simulink model "model_podstawowy_swingup_2015a"  (R2019b)
settings: Solver=ode45  StartTime=0.0  StopTime=15  RelTol=1e-3
undefined symbols (not defined in the file): g, J, K_reg, L, m, M, Q2, theta, x, x_konc, x_pocz
libraries: simulink x8
settings Model: Creator=maelstro  LastModifiedBy=Czarek
settings OptimizationCC: LifeSpan=inf
settings DebuggingCC: SFExecutionAtInitializationDiag=none  ArithmeticOperatorsInVariantConditions=warning
settings HardwareCC: ProdBitPerSizeT=32  ProdBitPerPtrDiffT=32  ProdWordSize=32  ProdHWDeviceType=Specified
settings SFSimCC: CustomCodeUndefinedFunction=UseInterfaceOnly
settings CodeAppCC: StateflowObjectComments=on

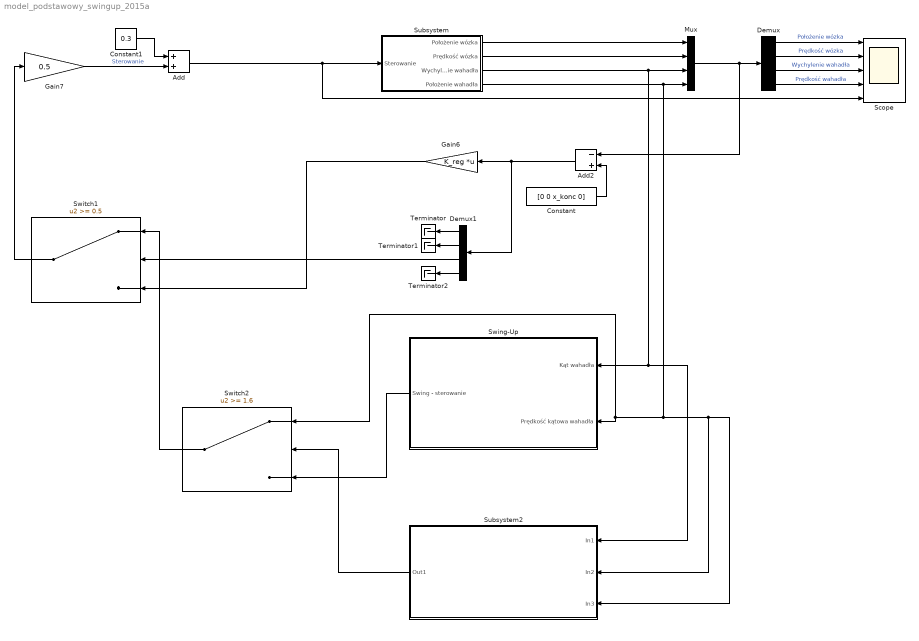
== system model_podstawowy_swingup_2015a ==
  Add : Sum
  Add2 : Sum  Inputs=-+
  Constant : Constant  Value=[0 0 x_konc 0]
  Constant1 : Constant  Value=0.3
  Demux : Demux
  Demux1 : Demux
  Gain6 : Gain  Gain=K_reg  Multiplication=Matrix(K*u)
  Gain7 : Gain  Gain=0.5
  Mux : Mux
  Scope : Scope  NumInputPorts=5
  Subsystem : Subsystem
  Subsystem2 : Subsystem
  Swing-Up : Subsystem
  Switch1 : Switch  Threshold=0.5
  Switch2 : Switch  Threshold=1.6
  Terminator : Terminator
  Terminator1 : Terminator
  Terminator2 : Terminator
  wires:
  Add2/1 -> Demux1/1, Gain6/1
  Mux/1 -> Demux/1, Add2/1
  Constant/1 -> Add2/2
  Subsystem/1(Położenie wózka) -> Mux/1
  Subsystem/2(Prędkość wózka) -> Mux/2
  Demux/1 -> Scope/1  "Położenie wózka"
  Demux/2 -> Scope/2  "Prędkość wózka"
  Demux/3 -> Scope/3  "Wychylenie wahadła"
  Demux/4 -> Scope/4  "Prędkość wahadła"
  Subsystem/4(Położenie wahadła) -> Switch2/1, Swing-Up/2(Prędkość kątowa wahadła), Subsystem2/3(In3), Subsystem2/2(In2), Mux/4
  Subsystem2/1(Out1) -> Switch2/2
  Switch2/1 -> Switch1/1
  Gain6/1 -> Switch1/3
  Subsystem/3(Wychylenie wahadła) -> Swing-Up/1(Kąt wahadła), Subsystem2/1(In1), Mux/3
  Swing-Up/1(Swing - sterowanie) -> Switch2/3
  Demux1/4 -> Terminator2/1
  Demux1/2 -> Terminator1/1
  Demux1/1 -> Terminator/1
  Demux1/3 -> Switch1/2
  Switch1/1 -> Gain7/1
  Gain7/1 -> Add/2  "Sterowanie"
  Add/1 -> Scope/5, Subsystem/1(Sterowanie)
  Constant1/1 -> Add/1

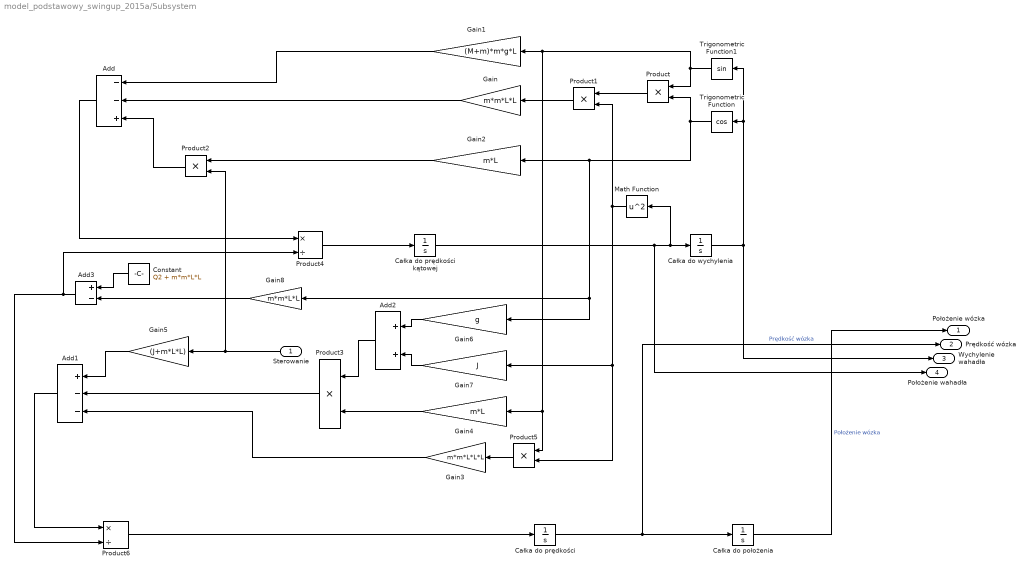
== system model_podstawowy_swingup_2015a/Subsystem ==
  Sterowanie : Inport
  Add : Sum  Inputs=--+
  Add1 : Sum  Inputs=+--
  Add2 : Sum
  Add3 : Sum  Inputs=+-
  Całka do położenia : Integrator
  Całka do prędkości : Integrator
  Całka do prędkości kątowej : Integrator
  Całka do wychylenia : Integrator  InitialCondition=x_pocz
  Constant : Constant  Value=Q2 + m*m*L*L
  Gain : Gain  Gain=m*m*L*L
  Gain1 : Gain  Gain=(M+m)*m*g*L
  Gain2 : Gain  Gain=m*L
  Gain3 : Gain  Gain=m*m*L*L*L
  Gain4 : Gain  Gain=m*L
  Gain5 : Gain  Gain=(J+m*L*L)
  Gain6 : Gain  Gain=g
  Gain7 : Gain  Gain=J
  Gain8 : Gain  Gain=m*m*L*L
  Math Function : Math  Operator=square  SaturateOnIntegerOverflow=on
  Product{,1..3,5} (5 alike) : Product
  Product4 : Product  Inputs=*/
  Product6 : Product  Inputs=*/
  Trigonometric Function : Trigonometry  Operator=cos
  Trigonometric Function1 : Trigonometry
  Położenie wózka : Outport
  Prędkość wózka : Outport  Port=2
  Wychylenie wahadła : Outport  Port=3
  Położenie wahadła : Outport  Port=4
  wires:
  Add/1 -> Product4/1
  Całka do prędkości/1 -> Prędkość wózka/1, Całka do położenia/1  "Prędkość wózka"
  Gain4/1 -> Product3/2
  Sterowanie/1 -> Product2/2, Gain5/1
  Product3/1 -> Add1/2
  Trigonometric Function/1 -> Gain8/1, Gain6/1, Gain2/1, Product/2
  Gain2/1 -> Product2/1
  Product1/1 -> Gain/1
  Całka do wychylenia/1 -> Wychylenie wahadła/1, Trigonometric Function1/1, Trigonometric Function/1
  Całka do położenia/1 -> Położenie wózka/1  "Położenie wózka"
  Add1/1 -> Product6/1
  Trigonometric Function1/1 -> Product/1, Product5/1, Gain4/1, Gain1/1
  Product4/1 -> Całka do prędkości kątowej/1
  Gain/1 -> Add/2
  Gain1/1 -> Add/1
  Product/1 -> Product1/1
  Product2/1 -> Add/3
  Gain3/1 -> Add1/3
  Całka do prędkości kątowej/1 -> Położenie wahadła/1, Math Function/1, Całka do wychylenia/1
  Gain5/1 -> Add1/1
  Math Function/1 -> Product1/2, Product5/2, Gain7/1
  Gain7/1 -> Add2/2
  Gain6/1 -> Add2/1
  Add2/1 -> Product3/1
  Product5/1 -> Gain3/1
  Product6/1 -> Całka do prędkości/1
  Add3/1 -> Product4/2, Product6/2
  Constant/1 -> Add3/1
  Gain8/1 -> Add3/2

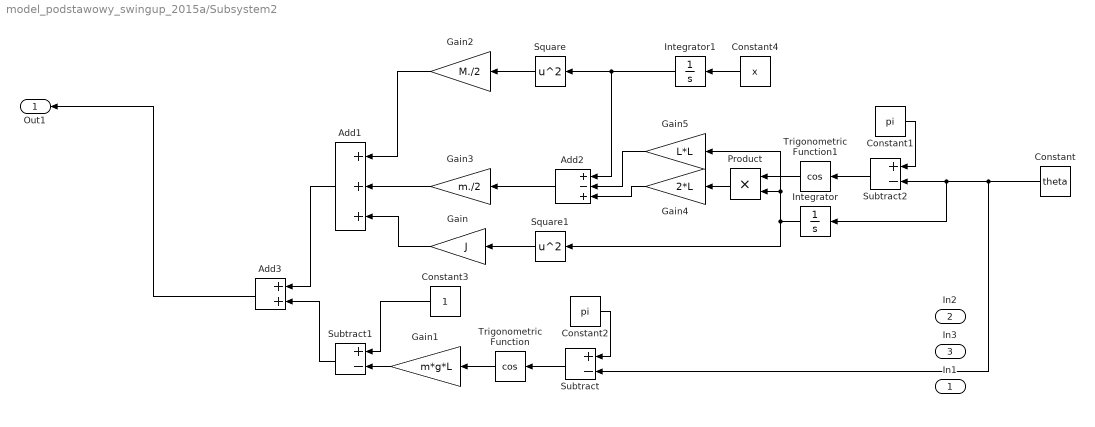
== system model_podstawowy_swingup_2015a/Subsystem2 ==
  In1 : Inport
  In2 : Inport  Port=2
  In3 : Inport  Port=3
  Add1 : Sum  Inputs=+++
  Add2 : Sum  Inputs=+-+
  Add3 : Sum
  Constant : Constant  Value=theta
  Constant1 : Constant  Value=pi
  Constant2 : Constant  Value=pi
  Constant3 : Constant
  Constant4 : Constant  Value=x
  Gain : Gain  Gain=J
  Gain1 : Gain  Gain=m*g*L
  Gain2 : Gain  Gain=M./2
  Gain3 : Gain  Gain=m./2
  Gain4 : Gain  Gain=2*L
  Gain5 : Gain  Gain=L*L
  Integrator : Integrator
  Integrator1 : Integrator
  Product : Product
  Square : Math  Operator=square  SignedPower=off  SaturateOnIntegerOverflow=on
  Square1 : Math  Operator=square  SignedPower=off  SaturateOnIntegerOverflow=on
  Subtract : Sum  Inputs=+-
  Subtract1 : Sum  Inputs=+-
  Subtract2 : Sum  Inputs=+-
  Trigonometric Function : Trigonometry  Operator=cos
  Trigonometric Function1 : Trigonometry  Operator=cos
  Out1 : Outport
  wires:
  Trigonometric Function/1 -> Gain1/1
  Subtract1/1 -> Add3/2
  Gain/1 -> Add1/3
  Constant2/1 -> Subtract/1
  Gain1/1 -> Subtract1/2
  Add3/1 -> Out1/1
  Square1/1 -> Gain/1
  Subtract/1 -> Trigonometric Function/1
  Constant3/1 -> Subtract1/1
  Gain2/1 -> Add1/1
  Square/1 -> Gain2/1
  Gain3/1 -> Add1/2
  Add2/1 -> Gain3/1
  Gain4/1 -> Add2/3
  Gain5/1 -> Add2/2
  Subtract2/1 -> Trigonometric Function1/1
  Constant1/1 -> Subtract2/1
  Constant/1 -> Subtract/2, Integrator/1, Subtract2/2
  Product/1 -> Gain4/1
  Trigonometric Function1/1 -> Product/1
  Integrator/1 -> Square1/1, Gain5/1, Product/2
  Integrator1/1 -> Add2/1, Square/1
  Constant4/1 -> Integrator1/1
  Add1/1 -> Add3/1

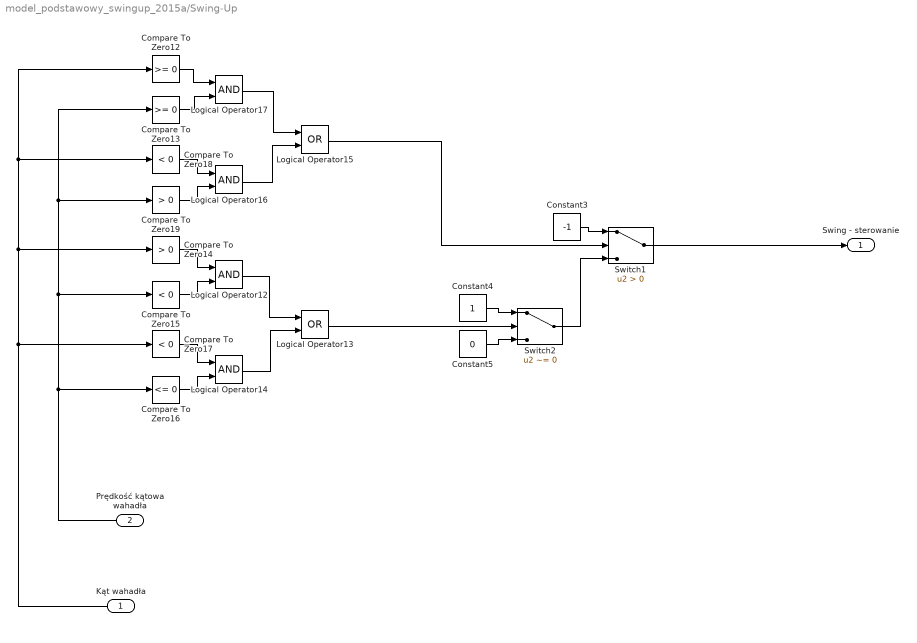
== system model_podstawowy_swingup_2015a/Swing-Up ==
  Kąt wahadła : Inport
  Prędkość kątowa wahadła : Inport  Port=2
  Compare To Zero12 : simulink/Logic and Bit Operations/Compare To Zero  relop=>=  OutDataTypeStr=uint8
  Compare To Zero13 : simulink/Logic and Bit Operations/Compare To Zero  relop=>=  OutDataTypeStr=uint8
  Compare To Zero14 : simulink/Logic and Bit Operations/Compare To Zero  relop=>  OutDataTypeStr=uint8
  Compare To Zero15 : simulink/Logic and Bit Operations/Compare To Zero  relop=<  OutDataTypeStr=uint8
  Compare To Zero16 : simulink/Logic and Bit Operations/Compare To Zero  relop=<=  OutDataTypeStr=uint8
  Compare To Zero17 : simulink/Logic and Bit Operations/Compare To Zero  relop=<  OutDataTypeStr=uint8
  Compare To Zero18 : simulink/Logic and Bit Operations/Compare To Zero  relop=<  OutDataTypeStr=uint8
  Compare To Zero19 : simulink/Logic and Bit Operations/Compare To Zero  relop=>  OutDataTypeStr=uint8
  Constant3 : Constant  Value=-1
  Constant4 : Constant
  Constant5 : Constant  Value=0
  Logical Operator{12,14,16..17} (4 alike) : Logic  AllPortsSameDT=off  OutDataTypeStr=boolean
  Logical Operator13 : Logic  Operator=OR  AllPortsSameDT=off  OutDataTypeStr=boolean
  Logical Operator15 : Logic  Operator=OR  AllPortsSameDT=off  OutDataTypeStr=boolean
  Switch1 : Switch  Criteria=u2 > Threshold
  Switch2 : Switch  Criteria=u2 ~= 0
  Swing - sterowanie : Outport
  wires:
  Prędkość kątowa wahadła/1 -> Compare To Zero15/1, Compare To Zero19/1, Compare To Zero13/1, Compare To Zero16/1
  Kąt wahadła/1 -> Compare To Zero17/1, Compare To Zero14/1, Compare To Zero18/1, Compare To Zero12/1
  Switch1/1 -> Swing - sterowanie/1
  Compare To Zero16/1 -> Logical Operator14/2
  Compare To Zero18/1 -> Logical Operator16/1
  Switch2/1 -> Switch1/3
  Logical Operator14/1 -> Logical Operator13/2
  Constant5/1 -> Switch2/3
  Logical Operator12/1 -> Logical Operator13/1
  Compare To Zero17/1 -> Logical Operator14/1
  Compare To Zero12/1 -> Logical Operator17/1
  Logical Operator16/1 -> Logical Operator15/2
  Compare To Zero14/1 -> Logical Operator12/1
  Constant4/1 -> Switch2/1
  Compare To Zero15/1 -> Logical Operator12/2
  Compare To Zero13/1 -> Logical Operator17/2
  Logical Operator17/1 -> Logical Operator15/1
  Logical Operator15/1 -> Switch1/2
  Constant3/1 -> Switch1/1
  Compare To Zero19/1 -> Logical Operator16/2
  Logical Operator13/1 -> Switch2/2
